simulink model "GearsetDefinition"  (R2018b)
settings: configuration reference "Physics" (kept outside this file)
model workspace (MAT data in the model file):
  m = 1000
undefined symbols (not defined in the file): POWTR__ENGINE__n_lb_rpm__1, POWTR__ENGINE__n_lb_rpm__2, POWTR__ENGINE__n_lb_rpm__3, POWTR__ENGINE__n_lb_rpm__4, POWTR__ENGINE__n_lb_rpm__5, POWTR__ENGINE__n_lb_rpm__6, POWTR__TRANSMISSION__gear__1, POWTR__TRANSMISSION__gear__2, POWTR__TRANSMISSION__gear__3, POWTR__TRANSMISSION__gear__4, POWTR__TRANSMISSION__gear__5, POWTR__TRANSMISSION__gear__6, POWTR__TRANSMISSION__gear_efficiency__1, POWTR__TRANSMISSION__gear_efficiency__2, POWTR__TRANSMISSION__gear_efficiency__3, POWTR__TRANSMISSION__gear_efficiency__4, POWTR__TRANSMISSION__gear_efficiency__5, POWTR__TRANSMISSION__gear_efficiency__6, POWTR__TRANSMISSION__gear_ratio__1, POWTR__TRANSMISSION__gear_ratio__2, POWTR__TRANSMISSION__gear_ratio__3, POWTR__TRANSMISSION__gear_ratio__4, POWTR__TRANSMISSION__gear_ratio__5, POWTR__TRANSMISSION__gear_ratio__6
settings Model: DataDictionary=vehicleparameters_vehdynsim.sldd  PauseTimes=9.280  Creator=wischnewski  LastModifiedBy=ga25xiw

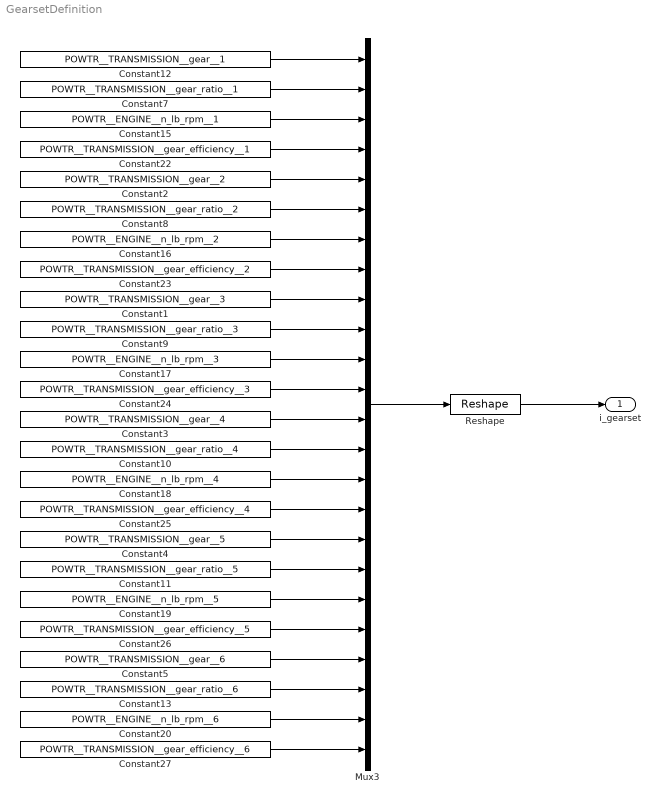
== system GearsetDefinition ==
  Constant1 : Constant  Value=POWTR__TRANSMISSION__gear__3
  Constant10 : Constant  Value=POWTR__TRANSMISSION__gear_ratio__4
  Constant11 : Constant  Value=POWTR__TRANSMISSION__gear_ratio__5
  Constant12 : Constant  Value=POWTR__TRANSMISSION__gear__1
  Constant13 : Constant  Value=POWTR__TRANSMISSION__gear_ratio__6
  Constant15 : Constant  Value=POWTR__ENGINE__n_lb_rpm__1
  Constant16 : Constant  Value=POWTR__ENGINE__n_lb_rpm__2
  Constant17 : Constant  Value=POWTR__ENGINE__n_lb_rpm__3
  Constant18 : Constant  Value=POWTR__ENGINE__n_lb_rpm__4
  Constant19 : Constant  Value=POWTR__ENGINE__n_lb_rpm__5
  Constant2 : Constant  Value=POWTR__TRANSMISSION__gear__2
  Constant20 : Constant  Value=POWTR__ENGINE__n_lb_rpm__6
  Constant22 : Constant  Value=POWTR__TRANSMISSION__gear_efficiency__1
  Constant23 : Constant  Value=POWTR__TRANSMISSION__gear_efficiency__2
  Constant24 : Constant  Value=POWTR__TRANSMISSION__gear_efficiency__3
  Constant25 : Constant  Value=POWTR__TRANSMISSION__gear_efficiency__4
  Constant26 : Constant  Value=POWTR__TRANSMISSION__gear_efficiency__5
  Constant27 : Constant  Value=POWTR__TRANSMISSION__gear_efficiency__6
  Constant3 : Constant  Value=POWTR__TRANSMISSION__gear__4
  Constant4 : Constant  Value=POWTR__TRANSMISSION__gear__5
  Constant5 : Constant  Value=POWTR__TRANSMISSION__gear__6
  Constant7 : Constant  Value=POWTR__TRANSMISSION__gear_ratio__1
  Constant8 : Constant  Value=POWTR__TRANSMISSION__gear_ratio__2
  Constant9 : Constant  Value=POWTR__TRANSMISSION__gear_ratio__3
  Mux3 : Mux  Inputs=24
  Reshape : Reshape  OutputDimensionality=Customize  OutputDimensions=[4,6]
  i_gearset : Outport
  wires:
  Constant2/1 -> Mux3/5
  Constant12/1 -> Mux3/1
  Constant22/1 -> Mux3/4
  Constant27/1 -> Mux3/24
  Mux3/1 -> Reshape/1
  Constant1/1 -> Mux3/9
  Constant18/1 -> Mux3/15
  Reshape/1 -> i_gearset/1
  Constant7/1 -> Mux3/2
  Constant4/1 -> Mux3/17
  Constant8/1 -> Mux3/6
  Constant11/1 -> Mux3/18
  Constant13/1 -> Mux3/22
  Constant15/1 -> Mux3/3
  Constant25/1 -> Mux3/16
  Constant10/1 -> Mux3/14
  Constant17/1 -> Mux3/11
  Constant9/1 -> Mux3/10
  Constant24/1 -> Mux3/12
  Constant5/1 -> Mux3/21
  Constant16/1 -> Mux3/7
  Constant26/1 -> Mux3/20
  Constant20/1 -> Mux3/23
  Constant3/1 -> Mux3/13
  Constant23/1 -> Mux3/8
  Constant19/1 -> Mux3/19
